simulink model "hydraulic_model"  (R2024a)
settings: Solver=ode23t  StartTime=0.0  StopTime=tEnd  FixedStep=1e-4  MaxStep=maxStep  RelTol=1e-2  AbsTol=1e-2
values from neighbouring files (symbols this model uses):
  boomHEArea = pi * (boomBoreDiameter/2)^2    (= 3117.24531052)    [init_model.m]
  boomREArea = pi * (boomBoreDiameter/2)^2 - pi*(boomRodDiameter/2)^2    (= 2410.38696347)    [init_model.m]
  swingDisplacement = 23.6    [init_model.m]
undefined symbols (not defined in the file or in its folder): ArmC, ArmR, AToTOrificeVector, BiPOrificeVector, BoomC, BoomR, boomValve, BToTOrificeVector, BucketC, BucketR, bucketValve, fluids, PToAOrificeVector, PToBOrificeVector, stickValve, SwingC, SwingR, swingValve, X, Y, Z
libraries: fl_lib x81, SimscapeFluids_lib x54, sm_lib x34, nesl_utility x29, spsFirstOrderFilterLib x4
(part 5 of 5)

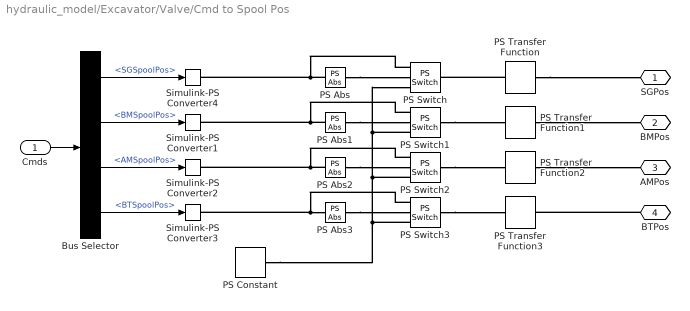
== system hydraulic_model/Excavator/Valve/Cmd to Spool Pos ==
  Cmds : Inport
  Bus Selector : BusSelector  OutputSignals=SGSpoolPos,BMSpoolPos,AMSpoolPos,BTSpoolPos
  PS Abs{,1..3} (4 alike) : fl_lib/Physical Signals/Nonlinear Operators/PS Abs
      settings: InternalSimscapePortConfiguration="{\"Bottom\":[],\"Left\":[{\"id\":\"I\",\"label\":\"\",\"type\":\"input\"}],\"Right\":[{\"id\":\"O\",\"label\":\"\",\"type\":\"output\"}],\"Top\":[]}"
  PS Constant : fl_lib/Physical Signals/Sources/PS Constant  constant=0.1 mm
  PS Switch{,1..3} (4 alike) : fl_lib/Physical Signals/Nonlinear Operators/PS Switch  Threshold=0.1 mm
      settings: InternalSimscapePortConfiguration="{\"Bottom\":[],\"Left\":[{\"id\":\"I1\",\"label\":\"\",\"type\":\"input\"},{\"id\":\"I2\",\"label\":\"\",\"type\":\"input\"},{\"id\":\"I3\",\"label\":\"\",\"type\":\"input\"}],\"Right\":[{\"id\":\"O\",\"label\":\"\",\"type\":\"output\"}],\"Top\":[]}"
  PS Transfer Function{,1..3} (4 alike) : fl_lib/Physical Signals/Linear Operators/PS Transfer Function  transfer_function_type=foundation.enum.transfer_function_type.lag  T=0.01 s  T1=2 s  T2=1 s  reset_method=foundation.enum.IntegratorResetSpec.None  initial_condition_spec=foundation.enum.IntegratorICSpec.Internal  y0=0 mm
      settings: InternalSimscapePortConfiguration="{\"Bottom\":[],\"Left\":[{\"id\":\"U\",\"label\":\"\",\"type\":\"input\"}],\"Right\":[{\"id\":\"Y\",\"label\":\"\",\"type\":\"output\"}],\"Top\":[]}"
  Simulink-PS Converter{1..4} (4 alike) : nesl_utility/Simulink-PS Converter  PhysicalDomain=network_engine_domain  SubClassName=ps_input  LeftPortType=input  RightPortType=output  PseudoPeriodic=off  Frequencies=[]  NoiseDistribution=none  NoiseParameters=[]  Unit=mm  AffineConversion=off  FilteringAndDerivatives=filter  SimscapeFilterOrder=1  InputFilterTimeConstant=0.01  UdotUserProvided=0
  SGPos : PMIOPort  Side=Right
  BMPos : PMIOPort  Port=2  Side=Right
  AMPos : PMIOPort  Port=3  Side=Right
  BTPos : PMIOPort  Port=4  Side=Right
  wires:
  Bus Selector/3 -> Simulink-PS Converter2/1  "<AMSpoolPos>"
  Bus Selector/1 -> Simulink-PS Converter4/1  "<SGSpoolPos>"
  Bus Selector/4 -> Simulink-PS Converter3/1  "<BTSpoolPos>"
  Bus Selector/2 -> Simulink-PS Converter1/1  "<BMSpoolPos>"
  Cmds/1 -> Bus Selector/1
  connections:
  PS Constant/RConn1 -- PS Switch/LConn3 -- PS Switch1/LConn3 -- PS Switch2/LConn3 -- PS Switch3/LConn3
  PS Switch/LConn1 -- Simulink-PS Converter4/RConn1 -- PS Abs/LConn1
  PS Abs2/LConn1 -- Simulink-PS Converter2/RConn1 -- PS Switch2/LConn1
  PS Abs/RConn1 -- PS Switch/LConn2
  PS Abs1/RConn1 -- PS Switch1/LConn2
  PS Abs2/RConn1 -- PS Switch2/LConn2
  PS Abs3/RConn1 -- PS Switch3/LConn2
  PS Abs1/LConn1 -- Simulink-PS Converter1/RConn1 -- PS Switch1/LConn1
  PS Switch3/LConn1 -- Simulink-PS Converter3/RConn1 -- PS Abs3/LConn1
  PS Transfer Function/RConn1 -- SGPos/RConn1
  PS Transfer Function/LConn1 -- PS Switch/RConn1
  PS Switch1/RConn1 -- PS Transfer Function1/LConn1
  PS Switch2/RConn1 -- PS Transfer Function2/LConn1
  PS Switch3/RConn1 -- PS Transfer Function3/LConn1
  PS Transfer Function1/RConn1 -- BMPos/RConn1
  PS Transfer Function2/RConn1 -- AMPos/RConn1
  BTPos/RConn1 -- PS Transfer Function3/RConn1

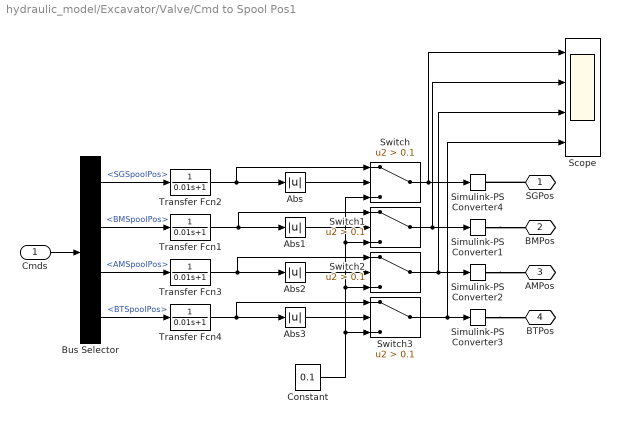
== system hydraulic_model/Excavator/Valve/Cmd to Spool Pos1 ==
  Cmds : Inport
  Abs{,1..3} (4 alike) : Abs  SaturateOnIntegerOverflow=off
  Bus Selector : BusSelector  OutputSignals=SGSpoolPos,BMSpoolPos,AMSpoolPos,BTSpoolPos
  Constant : Constant  Value=0.1
  Scope : Scope  NumInputPorts=4
  Simulink-PS Converter{1..4} (4 alike) : nesl_utility/Simulink-PS Converter  PhysicalDomain=network_engine_domain  SubClassName=ps_input  LeftPortType=input  RightPortType=output  PseudoPeriodic=off  Frequencies=[]  NoiseDistribution=none  NoiseParameters=[]  Unit=mm  AffineConversion=off  FilteringAndDerivatives=filter  SimscapeFilterOrder=1  InputFilterTimeConstant=0.01  UdotUserProvided=0
  Switch{,1..3} (4 alike) : Switch  Criteria=u2 > Threshold  Threshold=0.1  SaturateOnIntegerOverflow=off  InputSameDT=off
  Transfer Fcn{1..4} (4 alike) : TransferFcn  Denominator=[0.01 1]
  SGPos : PMIOPort  Side=Right
  BMPos : PMIOPort  Port=2  Side=Right
  AMPos : PMIOPort  Port=3  Side=Right
  BTPos : PMIOPort  Port=4  Side=Right
  wires:
  Bus Selector/3 -> Transfer Fcn3/1  "<AMSpoolPos>"
  Bus Selector/1 -> Transfer Fcn2/1  "<SGSpoolPos>"
  Bus Selector/4 -> Transfer Fcn4/1  "<BTSpoolPos>"
  Bus Selector/2 -> Transfer Fcn1/1  "<BMSpoolPos>"
  Cmds/1 -> Bus Selector/1
  Abs/1 -> Switch/2
  Abs1/1 -> Switch1/2
  Abs2/1 -> Switch2/2
  Abs3/1 -> Switch3/2
  Transfer Fcn2/1 -> Switch/1, Abs/1
  Transfer Fcn1/1 -> Switch1/1, Abs1/1
  Transfer Fcn3/1 -> Switch2/1, Abs2/1
  Transfer Fcn4/1 -> Switch3/1, Abs3/1
  Constant/1 -> Switch3/3, Switch2/3, Switch1/3, Switch/3
  Switch/1 -> Simulink-PS Converter4/1, Scope/1
  Switch1/1 -> Scope/2, Simulink-PS Converter1/1
  Switch2/1 -> Scope/3, Simulink-PS Converter2/1
  Switch3/1 -> Scope/4, Simulink-PS Converter3/1
  connections:
  SGPos/RConn1 -- Simulink-PS Converter4/RConn1
  Simulink-PS Converter1/RConn1 -- BMPos/RConn1
  Simulink-PS Converter2/RConn1 -- AMPos/RConn1
  Simulink-PS Converter3/RConn1 -- BTPos/RConn1

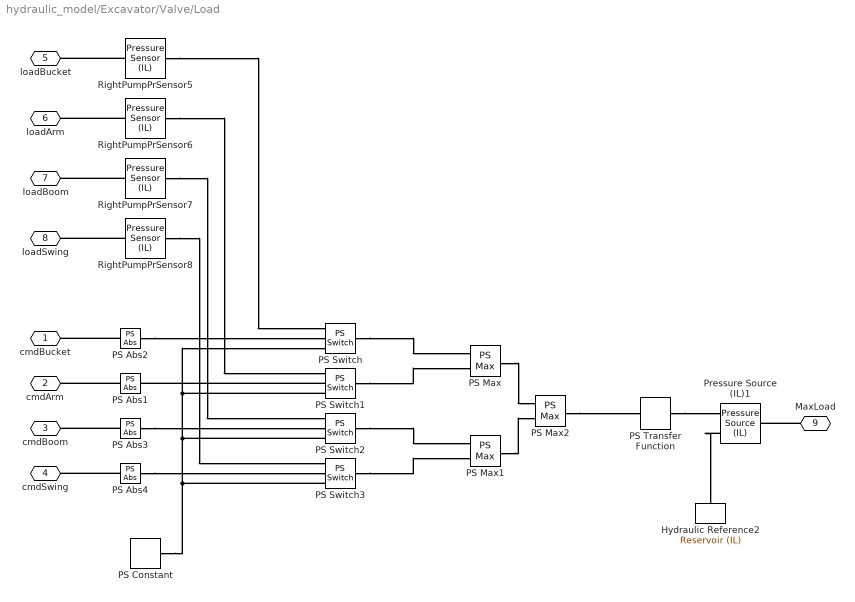
== system hydraulic_model/Excavator/Valve/Load ==
  Hydraulic Reference2 : fl_lib/Isothermal Liquid/Elements/Reservoir (IL)  reservoir_type=foundation.enum.constant_controlled.constant  pressure_spec=foundation.enum.pressure_spec.specified  reservoir_pressure=0.01 bar
  PS Abs{1..4} (4 alike) : fl_lib/Physical Signals/Nonlinear Operators/PS Abs
      settings: InternalSimscapePortConfiguration="{\"Bottom\":[],\"Left\":[{\"id\":\"I\",\"label\":\"\",\"type\":\"input\"}],\"Right\":[{\"id\":\"O\",\"label\":\"\",\"type\":\"output\"}],\"Top\":[]}"
  PS Constant : fl_lib/Physical Signals/Sources/PS Constant  constant=2 bar
  PS Max : fl_lib/Physical Signals/Nonlinear Operators/PS Max
      settings: InternalSimscapePortConfiguration="{\"Bottom\":[],\"Left\":[{\"id\":\"I1\",\"label\":\"\",\"type\":\"input\"},{\"id\":\"I2\",\"label\":\"\",\"type\":\"input\"}],\"Right\":[{\"id\":\"O\",\"label\":\"\",\"type\":\"output\"}],\"Top\":[]}"
  PS Max1 : fl_lib/Physical Signals/Nonlinear Operators/PS Max
      settings: InternalSimscapePortConfiguration="{\"Bottom\":[],\"Left\":[{\"id\":\"I1\",\"label\":\"\",\"type\":\"input\"},{\"id\":\"I2\",\"label\":\"\",\"type\":\"input\"}],\"Right\":[{\"id\":\"O\",\"label\":\"\",\"type\":\"output\"}],\"Top\":[]}"
  PS Max2 : fl_lib/Physical Signals/Nonlinear Operators/PS Max
      settings: InternalSimscapePortConfiguration="{\"Bottom\":[],\"Left\":[{\"id\":\"I1\",\"label\":\"\",\"type\":\"input\"},{\"id\":\"I2\",\"label\":\"\",\"type\":\"input\"}],\"Right\":[{\"id\":\"O\",\"label\":\"\",\"type\":\"output\"}],\"Top\":[]}"
  PS Switch{,1..3} (4 alike) : fl_lib/Physical Signals/Nonlinear Operators/PS Switch  Threshold=0.1 mm
      settings: InternalSimscapePortConfiguration="{\"Bottom\":[],\"Left\":[{\"id\":\"I1\",\"label\":\"\",\"type\":\"input\"},{\"id\":\"I2\",\"label\":\"\",\"type\":\"input\"},{\"id\":\"I3\",\"label\":\"\",\"type\":\"input\"}],\"Right\":[{\"id\":\"O\",\"label\":\"\",\"type\":\"output\"}],\"Top\":[]}"
  PS Transfer Function : fl_lib/Physical Signals/Linear Operators/PS Transfer Function  transfer_function_type=foundation.enum.transfer_function_type.lag  T=0.001 s  T1=2 s  T2=1 s  reset_method=foundation.enum.IntegratorResetSpec.None  initial_condition_spec=foundation.enum.IntegratorICSpec.Internal  y0=1.3 bar
      settings: InternalSimscapePortConfiguration="{\"Bottom\":[],\"Left\":[{\"id\":\"U\",\"label\":\"\",\"type\":\"input\"}],\"Right\":[{\"id\":\"Y\",\"label\":\"\",\"type\":\"output\"}],\"Top\":[]}"
  Pressure Source (IL)1 : fl_lib/Isothermal Liquid/Sources/Pressure Source (IL)  source_type=foundation.enum.constant_controlled.controlled  pressure_differential=0 MPa
      settings: InternalSimscapePortConfiguration="{\"Bottom\":[],\"Left\":[{\"id\":\"A\",\"label\":\"A\",\"type\":\"foundation.isothermal_liquid.isothermal_liquid\"},{\"id\":\"P\",\"label\":\"P\",\"type\":\"input\"}],\"Right\":[{\"id\":\"B\",\"label\":\"B\",\"type\":\"foundation.isothermal_liquid.isothermal_liquid\"}],\"Top\":[]}"
  RightPumpPrSensor{5..8} (4 alike) : fl_lib/Isothermal Liquid/Sensors/Pressure Sensor (IL)  pressure_measure=foundation.enum.pressure_measure.absolute
      settings: InternalSimscapePortConfiguration="{\"Bottom\":[],\"Left\":[{\"id\":\"A\",\"label\":\"A\",\"type\":\"foundation.isothermal_liquid.isothermal_liquid\"}],\"Right\":[{\"id\":\"Pa\",\"label\":\"Pa\",\"type\":\"output\"}],\"Top\":[]}"
  " cmdBucket" : PMIOPort  Side=Left
  " cmdArm" : PMIOPort  Port=2  Side=Left
  " cmdBoom" : PMIOPort  Port=3  Side=Left
  " cmdSwing" : PMIOPort  Port=4  Side=Left
  " loadBucket" : PMIOPort  Port=5  Side=Left
  " loadArm" : PMIOPort  Port=6  Side=Left
  " loadBoom" : PMIOPort  Port=7  Side=Left
  " loadSwing" : PMIOPort  Port=8  Side=Left
  MaxLoad : PMIOPort  Port=9  Side=Right
  connections:
  PS Transfer Function/RConn1 -- Pressure Source (IL)1/LConn2
  MaxLoad/RConn1 -- Pressure Source (IL)1/RConn1
  Pressure Source (IL)1/LConn1 -- Hydraulic Reference2/LConn1
  PS Max/RConn1 -- PS Max2/LConn1
  PS Max1/RConn1 -- PS Max2/LConn2
  RightPumpPrSensor8/LConn1 -- " loadSwing"/RConn1
  RightPumpPrSensor6/LConn1 -- " loadArm"/RConn1
  RightPumpPrSensor7/LConn1 -- " loadBoom"/RConn1
  RightPumpPrSensor5/LConn1 -- " loadBucket"/RConn1
  PS Abs2/RConn1 -- PS Switch/LConn2
  PS Abs3/RConn1 -- PS Switch2/LConn2
  PS Abs1/LConn1 -- " cmdArm"/RConn1
  PS Abs4/RConn1 -- PS Switch3/LConn2
  PS Constant/RConn1 -- PS Switch3/LConn3 -- PS Switch2/LConn3 -- PS Switch1/LConn3 -- PS Switch/LConn3
  RightPumpPrSensor5/RConn1 -- PS Switch/LConn1
  RightPumpPrSensor6/RConn1 -- PS Switch1/LConn1
  RightPumpPrSensor7/RConn1 -- PS Switch2/LConn1
  RightPumpPrSensor8/RConn1 -- PS Switch3/LConn1
  PS Switch/RConn1 -- PS Max/LConn1
  PS Switch1/RConn1 -- PS Max/LConn2
  PS Switch2/RConn1 -- PS Max1/LConn1
  PS Switch3/RConn1 -- PS Max1/LConn2
  PS Max2/RConn1 -- PS Transfer Function/LConn1
  PS Abs2/LConn1 -- " cmdBucket"/RConn1
  PS Switch1/LConn2 -- PS Abs1/RConn1
  PS Abs3/LConn1 -- " cmdBoom"/RConn1
  PS Abs4/LConn1 -- " cmdSwing"/RConn1

== system hydraulic_model/Excavator/Valve/Swing Valve ==
  AtoT : SimscapeFluids_lib/Isothermal Liquid/Valves & Orifices/Orifices/Orifice (IL)  orifice_type=foundation.enum.constant_variable.variable  constant_orifice_spec=fluids.isothermal_liquid.valves_orifices.orifices.enum.constant_orifice_spec.area  variable_orifice_spec=fluids.isothermal_liquid.valves_orifices.orifices.enum.orifice_spec.table1D_area_opening  orifice_area_constant=1e-3 m^2  p_diff_TLU_constant=[-4, -3, -2, -1, -.5, 0, .5, 1, 2, 3, 4] MPa  vol_flow_TLU_constant=[-2.44, -2.12, -1.68, -1.22, -.84, 0, .85, 1.21, 1.7, 2.09, 2.41] .* 1e-3 m^3/s  S_min=1e-10 m  del_S=0.005 m  open_orientation=fluids.isothermal_liquid.valves_orifices.orifices.enum.orifice_orientation.positive  area_max=0.5e-4 m^2  area_leak=1e-12 m^2  S_TLU=valveData.spoolPosVector mm  orifice_area_TLU=valveData.AtoTOrificeAreaVector mm^2  area=inf m^2  Cd=0.7  Re_c=150  smoothing_factor=0  pressure_recovery=simscape.enum.onoff.off  S_vol_flow_TLU=AToTOrificeVector - 1000*(0) mm  p_diff_TLU=[-10000000, -5000000, -2000000, 2000000, 5000000, 10000000] Pa  vol_flow_TLU=[-1e-07, -7.0711e-08, -4.4721e-08, 4.4721e-08, 7.0711e-08, 1e-07; -2.0352e-05, -1.4391e-05, -9.1017e-06, 9.1017e-06, 1.4391e-05, 2.0352e-05; -.0040736, -.0028805, -.0018218, .0018218, .0028805, .0040736; -.011438, -.0080879, -.0051152, .0051152, .0080879, .011438; -.034356, -.024293, -.015364, .015364, .024293, .034356] m^3/s  enable_faults=simscape.enum.onoff.off  fault_action=fluids.enum.FaultOpening.Closed
      settings: InternalSimscapePortConfiguration="{\"Bottom\":[],\"Left\":[{\"id\":\"A\",\"label\":\"A\",\"type\":\"foundation.isothermal_liquid.isothermal_liquid\"},{\"id\":\"S\",\"label\":\"S\",\"type\":\"input\"}],\"Right\":[{\"id\":\"B\",\"label\":\"B\",\"type\":\"foundation.isothermal_liquid.isothermal_liquid\"}],\"Top\":[]}"
  BiPOrifice : SimscapeFluids_lib/Isothermal Liquid/Valves & Orifices/Orifices/Orifice (IL)  orifice_type=foundation.enum.constant_variable.variable  constant_orifice_spec=fluids.isothermal_liquid.valves_orifices.orifices.enum.constant_orifice_spec.area  variable_orifice_spec=fluids.isothermal_liquid.valves_orifices.orifices.enum.orifice_spec.table1D_area_opening  orifice_area_constant=1e-3 m^2  p_diff_TLU_constant=[-4, -3, -2, -1, -.5, 0, .5, 1, 2, 3, 4] MPa  vol_flow_TLU_constant=[-2.44, -2.12, -1.68, -1.22, -.84, 0, .85, 1.21, 1.7, 2.09, 2.41] .* 1e-3 m^3/s  S_min=1e-10 m  del_S=0.005 m  open_orientation=fluids.isothermal_liquid.valves_orifices.orifices.enum.orifice_orientation.positive  area_max=0.5e-4 m^2  area_leak=1e-12 m^2  S_TLU=valveData.spoolPosVector mm  orifice_area_TLU=valveData.BiPOrificeAreaVector mm^2  area=inf m^2  Cd=0.7  Re_c=150  smoothing_factor=0  pressure_recovery=simscape.enum.onoff.off  S_vol_flow_TLU=BiPOrificeVector - 1000*(0) mm  p_diff_TLU=[-10000000, -5000000, -2000000, 2000000, 5000000, 10000000] Pa  vol_flow_TLU=[-1e-07, -7.0711e-08, -4.4721e-08, 4.4721e-08, 7.0711e-08, 1e-07; -2.0352e-05, -1.4391e-05, -9.1017e-06, 9.1017e-06, 1.4391e-05, 2.0352e-05; -.0040736, -.0028805, -.0018218, .0018218, .0028805, .0040736; -.011438, -.0080879, -.0051152, .0051152, .0080879, .011438; -.034356, -.024293, -.015364, .015364, .024293, .034356] m^3/s  enable_faults=simscape.enum.onoff.off  fault_action=fluids.enum.FaultOpening.Closed
      settings: InternalSimscapePortConfiguration="{\"Bottom\":[],\"Left\":[{\"id\":\"A\",\"label\":\"A\",\"type\":\"foundation.isothermal_liquid.isothermal_liquid\"},{\"id\":\"S\",\"label\":\"S\",\"type\":\"input\"}],\"Right\":[{\"id\":\"B\",\"label\":\"B\",\"type\":\"foundation.isothermal_liquid.isothermal_liquid\"}],\"Top\":[]}"
  BtoT : SimscapeFluids_lib/Isothermal Liquid/Valves & Orifices/Orifices/Orifice (IL)  orifice_type=foundation.enum.constant_variable.variable  constant_orifice_spec=fluids.isothermal_liquid.valves_orifices.orifices.enum.constant_orifice_spec.area  variable_orifice_spec=fluids.isothermal_liquid.valves_orifices.orifices.enum.orifice_spec.table1D_area_opening  orifice_area_constant=1e-3 m^2  p_diff_TLU_constant=[-4, -3, -2, -1, -.5, 0, .5, 1, 2, 3, 4] MPa  vol_flow_TLU_constant=[-2.44, -2.12, -1.68, -1.22, -.84, 0, .85, 1.21, 1.7, 2.09, 2.41] .* 1e-3 m^3/s  S_min=1e-10 m  del_S=0.005 m  open_orientation=fluids.isothermal_liquid.valves_orifices.orifices.enum.orifice_orientation.positive  area_max=0.5e-4 m^2  area_leak=1e-12 m^2  S_TLU=valveData.spoolPosVector mm  orifice_area_TLU=valveData.BtoTOrificeAreaVector mm^2  area=inf m^2  Cd=0.7  Re_c=150  smoothing_factor=0  pressure_recovery=simscape.enum.onoff.off  S_vol_flow_TLU=BToTOrificeVector - 1000*(0) mm  p_diff_TLU=[-10000000, -5000000, -2000000, 2000000, 5000000, 10000000] Pa  vol_flow_TLU=[-1e-07, -7.0711e-08, -4.4721e-08, 4.4721e-08, 7.0711e-08, 1e-07; -2.0352e-05, -1.4391e-05, -9.1017e-06, 9.1017e-06, 1.4391e-05, 2.0352e-05; -.0040736, -.0028805, -.0018218, .0018218, .0028805, .0040736; -.011438, -.0080879, -.0051152, .0051152, .0080879, .011438; -.034356, -.024293, -.015364, .015364, .024293, .034356] m^3/s  enable_faults=simscape.enum.onoff.off  fault_action=fluids.enum.FaultOpening.Closed
      settings: InternalSimscapePortConfiguration="{\"Bottom\":[],\"Left\":[{\"id\":\"A\",\"label\":\"A\",\"type\":\"foundation.isothermal_liquid.isothermal_liquid\"},{\"id\":\"S\",\"label\":\"S\",\"type\":\"input\"}],\"Right\":[{\"id\":\"B\",\"label\":\"B\",\"type\":\"foundation.isothermal_liquid.isothermal_liquid\"}],\"Top\":[]}"
  PS Abs : fl_lib/Physical Signals/Nonlinear Operators/PS Abs
      settings: InternalSimscapePortConfiguration="{\"Bottom\":[],\"Left\":[{\"id\":\"I\",\"label\":\"\",\"type\":\"input\"}],\"Right\":[{\"id\":\"O\",\"label\":\"\",\"type\":\"output\"}],\"Top\":[]}"
  PS Gain2 : fl_lib/Physical Signals/Functions/PS Gain  gain=-1
  Pressure Compensator Valve (IL) : SimscapeFluids_lib/Isothermal Liquid/Valves & Orifices/Pressure Control Valves/Pressure Compensator Valve (IL)  valve_spec=fluids.isothermal_liquid.valves_orifices.enum.closed_open.open  set_pressure_spec=foundation.enum.constant_controlled.constant  opening_spec=fluids.isothermal_liquid.valves_orifices.enum.opening_spec.linear  p_set_differential=0 MPa  p_range=1.5 bar  area_max=1e-4 m^2  area_leak=1e-10 m^2  p_diff_reducing_TLU=[0.2 : 0.2 : 1.2] MPa  valve_area_reducing_TLU=[1e-05, 8e-06, 6e-06, 4e-06, 2e-06, 1e-10] m^2  p_diff_relief_TLU=[0.2 : 0.2 : 1.2] MPa  valve_area_relief_TLU=[1e-10, 2e-06, 4e-06, 6e-06, 8e-06, 1e-05] m^2  area=inf m^2  Cd=0.7  Re_c=150  smoothing_factor=0.01  pressure_recovery=false  opening_dynamics=true  tau=0.01 s  enable_faults=simscape.enum.onoff.off  fault_type=fluids.enum.FaultOpening.Closed  faulted_specify=off  faulted_priority=High  faulted=0
      settings: InternalSimscapePortConfiguration="{\"Bottom\":[],\"Left\":[{\"id\":\"A\",\"label\":\"A\",\"type\":\"foundation.isothermal_liquid.isothermal_liquid\"}],\"Right\":[{\"id\":\"X\",\"label\":\"X\",\"type\":\"foundation.isothermal_liquid.isothermal_liquid\"},{\"id\":\"B\",\"label\":\"B\",\"type\":\"foundation.isothermal_liquid.isothermal_liquid\"},{\"id\":\"Y\",\"label\":\"Y\",\"type\":\"foundation.isothermal_liquid.isothermal_liquid\"}],\"Top\":[]}"
  PtoA : SimscapeFluids_lib/Isothermal Liquid/Valves & Orifices/Orifices/Orifice (IL)  orifice_type=foundation.enum.constant_variable.variable  constant_orifice_spec=fluids.isothermal_liquid.valves_orifices.orifices.enum.constant_orifice_spec.area  variable_orifice_spec=fluids.isothermal_liquid.valves_orifices.orifices.enum.orifice_spec.table1D_area_opening  orifice_area_constant=1e-3 m^2  p_diff_TLU_constant=[-4, -3, -2, -1, -.5, 0, .5, 1, 2, 3, 4] MPa  vol_flow_TLU_constant=[-2.44, -2.12, -1.68, -1.22, -.84, 0, .85, 1.21, 1.7, 2.09, 2.41] .* 1e-3 m^3/s  S_min=1e-10 m  del_S=0.005 m  open_orientation=fluids.isothermal_liquid.valves_orifices.orifices.enum.orifice_orientation.positive  area_max=0.5e-4 m^2  area_leak=1e-12 m^2  S_TLU=valveData.spoolPosVector mm  orifice_area_TLU=valveData.PtoAOrificeAreaVector mm^2  area=inf m^2  Cd=0.7  Re_c=150  smoothing_factor=0  pressure_recovery=simscape.enum.onoff.off  S_vol_flow_TLU=PToAOrificeVector - 1000*(0) mm  p_diff_TLU=[-10000000, -5000000, -2000000, 2000000, 5000000, 10000000] Pa  vol_flow_TLU=[-1e-07, -7.0711e-08, -4.4721e-08, 4.4721e-08, 7.0711e-08, 1e-07; -2.0352e-05, -1.4391e-05, -9.1017e-06, 9.1017e-06, 1.4391e-05, 2.0352e-05; -.0040736, -.0028805, -.0018218, .0018218, .0028805, .0040736; -.011438, -.0080879, -.0051152, .0051152, .0080879, .011438; -.034356, -.024293, -.015364, .015364, .024293, .034356] m^3/s  enable_faults=simscape.enum.onoff.off  fault_action=fluids.enum.FaultOpening.Closed
      settings: InternalSimscapePortConfiguration="{\"Bottom\":[],\"Left\":[{\"id\":\"A\",\"label\":\"A\",\"type\":\"foundation.isothermal_liquid.isothermal_liquid\"},{\"id\":\"S\",\"label\":\"S\",\"type\":\"input\"}],\"Right\":[{\"id\":\"B\",\"label\":\"B\",\"type\":\"foundation.isothermal_liquid.isothermal_liquid\"}],\"Top\":[]}"
  PtoB : SimscapeFluids_lib/Isothermal Liquid/Valves & Orifices/Orifices/Orifice (IL)  orifice_type=foundation.enum.constant_variable.variable  constant_orifice_spec=fluids.isothermal_liquid.valves_orifices.orifices.enum.constant_orifice_spec.area  variable_orifice_spec=fluids.isothermal_liquid.valves_orifices.orifices.enum.orifice_spec.table1D_area_opening  orifice_area_constant=1e-3 m^2  p_diff_TLU_constant=[-4, -3, -2, -1, -.5, 0, .5, 1, 2, 3, 4] MPa  vol_flow_TLU_constant=[-2.44, -2.12, -1.68, -1.22, -.84, 0, .85, 1.21, 1.7, 2.09, 2.41] .* 1e-3 m^3/s  S_min=1e-10 m  del_S=0.005 m  open_orientation=fluids.isothermal_liquid.valves_orifices.orifices.enum.orifice_orientation.positive  area_max=0.5e-4 m^2  area_leak=1e-12 m^2  S_TLU=valveData.spoolPosVector mm  orifice_area_TLU=valveData.PtoBOrificeAreaVector mm^2  area=inf m^2  Cd=0.7  Re_c=150  smoothing_factor=0  pressure_recovery=simscape.enum.onoff.off  S_vol_flow_TLU=PToBOrificeVector - 1000*(0) mm  p_diff_TLU=[-10000000, -5000000, -2000000, 2000000, 5000000, 10000000] Pa  vol_flow_TLU=[-1e-07, -7.0711e-08, -4.4721e-08, 4.4721e-08, 7.0711e-08, 1e-07; -2.0352e-05, -1.4391e-05, -9.1017e-06, 9.1017e-06, 1.4391e-05, 2.0352e-05; -.0040736, -.0028805, -.0018218, .0018218, .0028805, .0040736; -.011438, -.0080879, -.0051152, .0051152, .0080879, .011438; -.034356, -.024293, -.015364, .015364, .024293, .034356] m^3/s  enable_faults=simscape.enum.onoff.off  fault_action=fluids.enum.FaultOpening.Closed
      settings: InternalSimscapePortConfiguration="{\"Bottom\":[],\"Left\":[{\"id\":\"A\",\"label\":\"A\",\"type\":\"foundation.isothermal_liquid.isothermal_liquid\"},{\"id\":\"S\",\"label\":\"S\",\"type\":\"input\"}],\"Right\":[{\"id\":\"B\",\"label\":\"B\",\"type\":\"foundation.isothermal_liquid.isothermal_liquid\"}],\"Top\":[]}"
  S : PMIOPort  Side=Left
  T : PMIOPort  Port=2  Side=Left
  A : PMIOPort  Port=3  Side=Right
  B : PMIOPort  Port=4  Side=Right
  P : PMIOPort  Port=5  Side=Left
  MaxLoad : PMIOPort  Port=6  Side=Left
  LoadSG : PMIOPort  Port=7  Side=Right
  connections:
  BtoT/LConn2 -- PtoA/LConn2 -- PS Gain2/LConn1 -- S/RConn1 -- PS Abs/LConn1
  BiPOrifice/LConn2 -- PS Abs/RConn1
  BtoT/RConn1 -- T/RConn1 -- AtoT/RConn1
  PtoA/RConn1 -- A/RConn1 -- AtoT/LConn1
  PtoA/LConn1 -- Pressure Compensator Valve (IL)/RConn2 -- LoadSG/RConn1 -- PtoB/LConn1
  PtoB/RConn1 -- B/RConn1 -- BtoT/LConn1
  P/RConn1 -- BiPOrifice/LConn1
  Pressure Compensator Valve (IL)/LConn1 -- BiPOrifice/RConn1 -- Pressure Compensator Valve (IL)/RConn3
  Pressure Compensator Valve (IL)/RConn1 -- MaxLoad/RConn1
  PS Gain2/RConn1 -- PtoB/LConn2 -- AtoT/LConn2

== matlab function hydraulic_model/Excavator/Timer/MATLAB Function ==
  data: current_time input; Tmp input; time_differ output
function time_differ = fcn(current_time, Tmp)
current_time = round(1e4 * current_time);
Tmp = round(1e4 * Tmp);

time_differ = (current_time - Tmp) * 1e-4;
